simulink model "zad3simulink"  (R2023a)
settings: Solver=VariableStepAuto  StartTime=0.0  StopTime=10  RelTol=1e-3
values from neighbouring files (symbols this model uses):
  Gz = c2d(Gs,T,'zoh')    [zad1.m]
  T = 0.5    [zad1.m]    (also in zad4.mat)
settings Model: Creator=pkutyl  LastModifiedBy=pkutyl

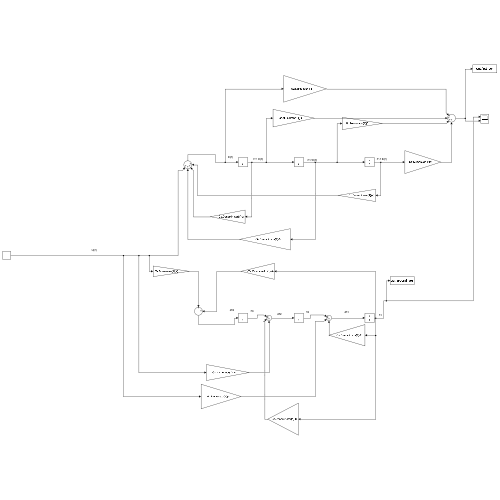
[thumbnail: Simulink's stored preview of the top-level diagram]
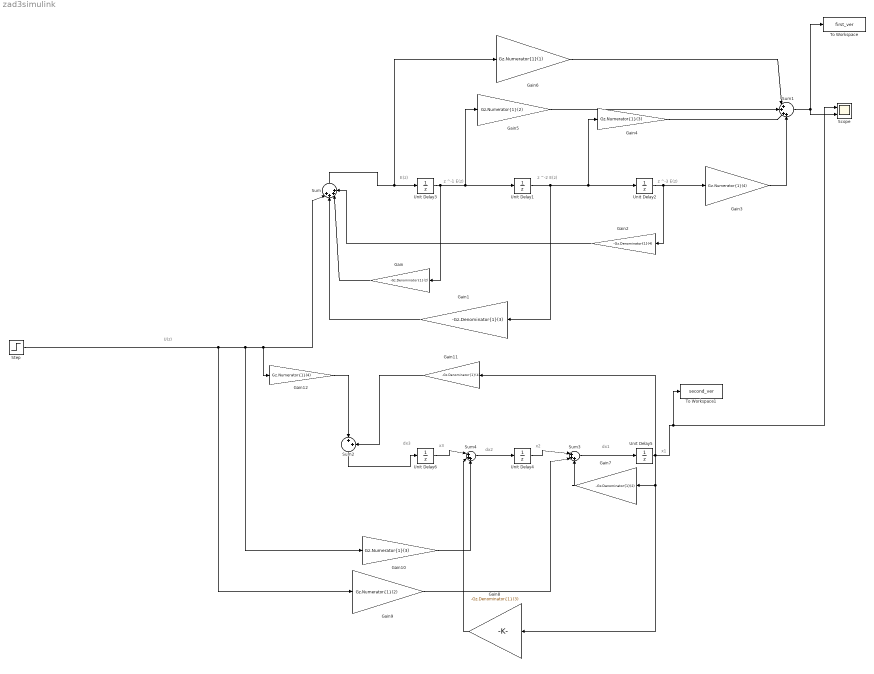
== system zad3simulink ==
  note: E(z)
  note: z ^-1 E(z)
  note: U(z)
  note: z ^-2 E(z)
  note: z ^-3 E(z)
  note: dx3
  note: dx2
  note: x1
  note: x2
  note: x3
  note: dx1
  Gain : Gain  Gain=-Gz.Denominator{1}(2)
  Gain1 : Gain  Gain=-Gz.Denominator{1}(3)
  Gain10 : Gain  Gain=Gz.Numerator{1}(3)
  Gain11 : Gain  Gain=-Gz.Denominator{1}(4)
  Gain12 : Gain  Gain=Gz.Numerator{1}(4)
  Gain2 : Gain  Gain=-Gz.Denominator{1}(4)
  Gain3 : Gain  Gain=Gz.Numerator{1}(4)
  Gain4 : Gain  Gain=Gz.Numerator{1}(3)
  Gain5 : Gain  Gain=Gz.Numerator{1}(2)
  Gain6 : Gain  Gain=Gz.Numerator{1}(1)
  Gain7 : Gain  Gain=-Gz.Denominator{1}(2)
  Gain8 : Gain  Gain=-Gz.Denominator{1}(3)
  Gain9 : Gain  Gain=Gz.Numerator{1}(2)
  Scope : Scope  NumInputPorts=2
  Step : Step  SampleTime=T
  Sum : Sum  Inputs=|++++
  Sum1 : Sum  Inputs=|++++
  Sum2 : Sum  Inputs=|++
  Sum3 : Sum  Inputs=|+++
  Sum4 : Sum  Inputs=|+++
  To Workspace : ToWorkspace  VariableName=first_ver  SaveFormat=Structure With Time  SampleTime=-1
  To Workspace1 : ToWorkspace  VariableName=second_ver  SaveFormat=Structure With Time  SampleTime=-1
  Unit Delay{1..6} (6 alike) : UnitDelay  SampleTime=T  HasFrameUpgradeWarning=on
  wires:
  Unit Delay1/1 -> Gain1/1, Gain4/1, Unit Delay2/1
  Sum/1 -> Unit Delay3/1, Gain6/1
  Step/1 -> Gain9/1, Gain10/1, Gain12/1, Sum/1
  Gain4/1 -> Sum1/3
  Unit Delay2/1 -> Gain2/1, Gain3/1
  Gain6/1 -> Sum1/1
  Gain3/1 -> Sum1/4
  Gain5/1 -> Sum1/2
  Gain2/1 -> Sum/4
  Sum1/1 -> To Workspace/1, Scope/2
  Gain1/1 -> Sum/2
  Gain/1 -> Sum/3
  Unit Delay3/1 -> Gain/1, Gain5/1, Unit Delay1/1
  Unit Delay6/1 -> Sum4/1
  Unit Delay4/1 -> Sum3/1
  Sum2/1 -> Unit Delay6/1
  Sum4/1 -> Unit Delay4/1
  Gain11/1 -> Sum2/2
  Gain9/1 -> Sum3/2
  Gain10/1 -> Sum4/3
  Gain12/1 -> Sum2/1
  Sum3/1 -> Unit Delay5/1
  Unit Delay5/1 -> Gain8/1, Gain7/1, To Workspace1/1, Scope/1, Gain11/1
  Gain8/1 -> Sum4/2
  Gain7/1 -> Sum3/3
